simulink model "Plant_N_LQR"  (R2017a)
settings: Solver=ode5  StartTime=0.0  StopTime=t  FixedStep=0.001  RelTol=1e-3  EnableMultiTasking=on
values from neighbouring files (symbols this model uses):
  K_LQR = -R1\B'*P    [Sc_H2LQR_R.m]
  t_stop = 35    [Sc_reference.m]    (also in pathdes.m = 50)
libraries: simulink x6
settings Model: Creator=GeoLee  LastModifiedBy=gmh_n
settings DataIOCC: LimitDataPoints=on  SaveFormat=Array
settings OptimizationCC: LifeSpan=inf
settings DebuggingCC: SFUnexpectedBacktrackingDiag=warning  SFNoUnconditionalDefaultTransitionDiag=warning  SFExecutionAtInitializationDiag=none
settings HardwareCC: ProdBitPerPointer=32  ProdBitPerSizeT=32  ProdBitPerPtrDiffT=32  ProdLargestAtomicFloat=None  ProdIntDivRoundTo=Undefined  ProdEndianess=Unspecified  ProdWordSize=32  ProdHWDeviceType=32-bit Generic
settings ModelReferenceCC: PropagateSignalLabelsOutOfModel=off
settings GRTTargetCC: TargetLangStandard=C89/C90 (ANSI)  GeneratePreprocessorConditionals=Disable all
settings ConfigComp: CovMetricSettings=dw  CovHtmlReporting=on  CovSaveCumulativeToWorkspaceVar=on  CovSaveSingleToWorkspaceVar=on  CovExternalEMLEnable=off

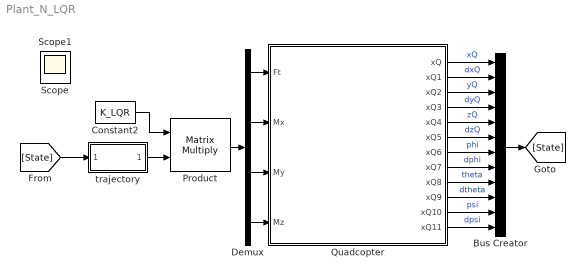
== system Plant_N_LQR ==
  Bus Creator : BusCreator  Inputs=12
  Constant2 : Constant  Value=K_LQR
  Demux : Demux
  Product : Product  Multiplication=Matrix(*)  RndMeth=Zero
  Quadcopter : Subsystem  mask(Single Quadcopter Plant){x0=0, y0=0, z0=0}
      mask prompts: x0 "Initial position of x (m)"; y0 "Initial position of y (m)"; z0 "Initial position of z (m)"
      mask help:
      | Attention:
      | the first input Ft is actually dF!
      mask Display:
      | image('Quad_pic.png');
      | port_label('input', 1, 'Ft');
      | port_label('input', 2, 'Mx');
      | port_label('input', 3, 'My');
      | port_label('input', 4, 'Mz');
      | port_label('output', 1, 'xQ');
      | port_label('output', 2, 'dxQ');
      | port_label('output', 3, 'yQ');
      | port_label('output', 4, 'dyQ');
      | port_label('output', 5, 'zQ');
      | port_label('output', 6, 'dzQ');
      | port_label('output', 7, 'phi');
      | port_label('output', 8, 'dphi');
      | port_label('output', 9, 'theta');
      | port_label('output', 10, 'dtheta');
      | port_label('output', 11, 'psi');
      | port_label('output', 12, 'dpsi');
  trajectory : Subsystem
  Scope : Scope
  Scope1 : Scope
  wires:
  Product/1 -> Demux/1
  [State] -> trajectory/1(State)
  trajectory/1(error) -> Product/2
  Quadcopter/6(xQ5) -> Bus Creator/6  "dzQ"
  Quadcopter/5(xQ4) -> Bus Creator/5  "zQ"
  Quadcopter/7(xQ6) -> Bus Creator/7  "phi"
  Quadcopter/4(xQ3) -> Bus Creator/4  "dyQ"
  Quadcopter/8(xQ7) -> Bus Creator/8  "dphi"
  Quadcopter/3(xQ2) -> Bus Creator/3  "yQ"
  Quadcopter/9(xQ8) -> Bus Creator/9  "theta"
  Quadcopter/2(xQ1) -> Bus Creator/2  "dxQ"
  Quadcopter/10(xQ9) -> Bus Creator/10  "dtheta"
  Quadcopter/11(xQ10) -> Bus Creator/11  "psi"
  Quadcopter/1(xQ) -> Bus Creator/1  "xQ"
  Quadcopter/12(xQ11) -> Bus Creator/12  "dpsi"
  Bus Creator/1 -> [State]
  Demux/1 -> Quadcopter/1(Ft)
  Demux/2 -> Quadcopter/2(Mx)
  Demux/4 -> Quadcopter/4(Mz)
  Demux/3 -> Quadcopter/3(My)
  Constant2/1 -> Product/1

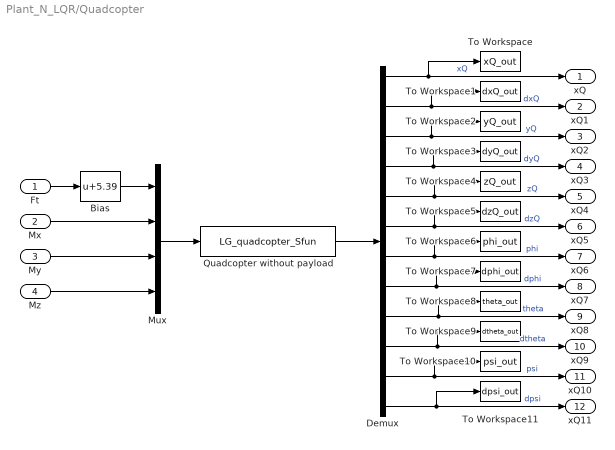
== system Plant_N_LQR/Quadcopter ==
  Ft : Inport
  Mx : Inport  Port=2
  My : Inport  Port=3
  Mz : Inport  Port=4
  Bias : Bias  Bias=5.39
  Demux : Demux  Outputs=12
  Mux : Mux
  Quadcopter without payload : S-Function  FunctionName=LG_quadcopter_Sfun  Parameters=x0,y0,z0  SFunctionDeploymentMode=off  EnableBusSupport=off
  To Workspace : ToWorkspace  VariableName=xQ_out  SampleTime=-1
  To Workspace1 : ToWorkspace  VariableName=dxQ_out  SampleTime=-1
  To Workspace10 : ToWorkspace  VariableName=psi_out  SampleTime=-1
  To Workspace11 : ToWorkspace  VariableName=dpsi_out  SampleTime=-1
  To Workspace2 : ToWorkspace  VariableName=yQ_out  SampleTime=-1
  To Workspace3 : ToWorkspace  VariableName=dyQ_out  SampleTime=-1
  To Workspace4 : ToWorkspace  VariableName=zQ_out  SampleTime=-1
  To Workspace5 : ToWorkspace  VariableName=dzQ_out  SampleTime=-1
  To Workspace6 : ToWorkspace  VariableName=phi_out  SampleTime=-1
  To Workspace7 : ToWorkspace  VariableName=dphi_out  SampleTime=-1
  To Workspace8 : ToWorkspace  VariableName=theta_out  SampleTime=-1
  To Workspace9 : ToWorkspace  VariableName=dtheta_out  SampleTime=-1
  xQ : Outport
  xQ1 : Outport  Port=2
  xQ2 : Outport  Port=3
  xQ3 : Outport  Port=4
  xQ4 : Outport  Port=5
  xQ5 : Outport  Port=6
  xQ6 : Outport  Port=7
  xQ7 : Outport  Port=8
  xQ8 : Outport  Port=9
  xQ9 : Outport  Port=10
  xQ10 : Outport  Port=11
  xQ11 : Outport  Port=12
  wires:
  Mux/1 -> Quadcopter without payload/1
  Ft/1 -> Bias/1
  Quadcopter without payload/1 -> Demux/1
  Mz/1 -> Mux/4
  Bias/1 -> Mux/1
  Demux/9 -> To Workspace8/1, xQ8/1  "theta"
  Demux/1 -> xQ/1, To Workspace/1  "xQ"
  Demux/7 -> xQ6/1, To Workspace6/1  "phi"
  Demux/11 -> xQ10/1, To Workspace10/1  "psi"
  Demux/4 -> xQ3/1, To Workspace3/1  "dyQ"
  Demux/2 -> xQ1/1, To Workspace1/1  "dxQ"
  Demux/3 -> xQ2/1, To Workspace2/1  "yQ"
  Demux/10 -> xQ9/1, To Workspace9/1  "dtheta"
  Demux/5 -> xQ4/1, To Workspace4/1  "zQ"
  Demux/8 -> xQ7/1, To Workspace7/1  "dphi"
  Demux/12 -> xQ11/1, To Workspace11/1  "dpsi"
  Demux/6 -> xQ5/1, To Workspace5/1  "dzQ"
  My/1 -> Mux/3
  Mx/1 -> Mux/2

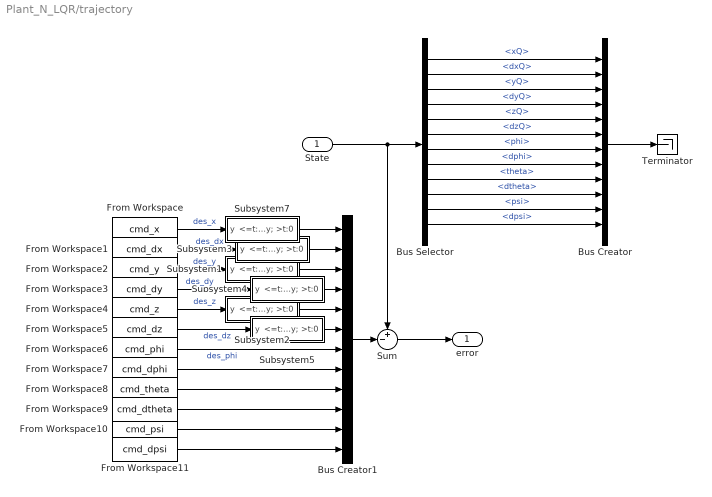
== system Plant_N_LQR/trajectory ==
  State : Inport
  Bus Creator : BusCreator  Inputs=12
  Bus Creator1 : BusCreator  Inputs=12
  Bus Selector : BusSelector  OutputSignals=xQ,dxQ,yQ,dyQ,zQ,dzQ,phi,dphi,theta,dtheta,psi,dpsi
  From Workspace : FromWorkspace  VariableName=cmd_x  SampleTime=0
  From Workspace1 : FromWorkspace  VariableName=cmd_dx  SampleTime=0
  From Workspace10 : FromWorkspace  VariableName=cmd_psi  SampleTime=0
  From Workspace11 : FromWorkspace  VariableName=cmd_dpsi  SampleTime=0
  From Workspace2 : FromWorkspace  VariableName=cmd_y  SampleTime=0
  From Workspace3 : FromWorkspace  VariableName=cmd_dy  SampleTime=0
  From Workspace4 : FromWorkspace  VariableName=cmd_z  SampleTime=0
  From Workspace5 : FromWorkspace  VariableName=cmd_dz  SampleTime=0
  From Workspace6 : FromWorkspace  VariableName=cmd_phi  SampleTime=0
  From Workspace7 : FromWorkspace  VariableName=cmd_dphi  SampleTime=0
  From Workspace8 : FromWorkspace  VariableName=cmd_theta  SampleTime=0
  From Workspace9 : FromWorkspace  VariableName=cmd_dtheta  SampleTime=0
  Subsystem1 : Subsystem
  Subsystem2 : Subsystem
  Subsystem3 : Subsystem
  Subsystem4 : Subsystem
  Subsystem5 : Subsystem
  Subsystem7 : Subsystem
  Sum : Sum  Inputs=+-|
  Terminator : Terminator
  error : Outport
  wires:
  Bus Selector/3 -> Bus Creator/3  "<yQ>"
  Bus Selector/9 -> Bus Creator/9  "<theta>"
  Bus Selector/10 -> Bus Creator/10  "<dtheta>"
  Bus Selector/7 -> Bus Creator/7  "<phi>"
  Bus Selector/2 -> Bus Creator/2  "<dxQ>"
  Bus Selector/8 -> Bus Creator/8  "<dphi>"
  Bus Selector/5 -> Bus Creator/5  "<zQ>"
  Bus Selector/4 -> Bus Creator/4  "<dyQ>"
  Bus Selector/11 -> Bus Creator/11  "<psi>"
  Bus Creator/1 -> Terminator/1
  Bus Selector/12 -> Bus Creator/12  "<dpsi>"
  Bus Selector/1 -> Bus Creator/1  "<xQ>"
  State/1 -> Bus Selector/1, Sum/1
  Bus Selector/6 -> Bus Creator/6  "<dzQ>"
  Bus Creator1/1 -> Sum/2
  From Workspace/1 -> Subsystem7/1(y)  "des_x"
  From Workspace1/1 -> Subsystem3/1(y)  "des_dx"
  From Workspace2/1 -> Subsystem1/1(y)  "des_y"
  From Workspace3/1 -> Subsystem4/1(y)  "des_dy"
  From Workspace4/1 -> Subsystem2/1(y)  "des_z"
  Sum/1 -> error/1
  From Workspace9/1 -> Bus Creator1/10
  From Workspace11/1 -> Bus Creator1/12
  From Workspace10/1 -> Bus Creator1/11
  From Workspace8/1 -> Bus Creator1/9
  From Workspace5/1 -> Subsystem5/1(y)  "des_dz"
  From Workspace6/1 -> Bus Creator1/7  "des_phi"
  From Workspace7/1 -> Bus Creator1/8
  Subsystem7/1(<=t:y; >t:0) -> Bus Creator1/1
  Subsystem1/1(<=t:y; >t:0) -> Bus Creator1/3
  Subsystem2/1(<=t:y; >t:0) -> Bus Creator1/5
  Subsystem3/1(<=t:y; >t:0) -> Bus Creator1/2
  Subsystem4/1(<=t:y; >t:0) -> Bus Creator1/4
  Subsystem5/1(<=t:y; >t:0) -> Bus Creator1/6

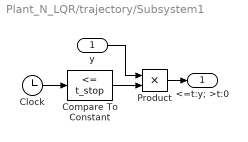
== system Plant_N_LQR/trajectory/Subsystem1 ==
  y : Inport
  Clock : Clock
  Compare To Constant : simulink/Logic and Bit Operations/Compare To Constant  relop=<=  const=t_stop  OutDataTypeStr=boolean
  Product : Product
  <=t:y; >t:0 : Outport
  wires:
  Compare To Constant/1 -> Product/2
  Product/1 -> <=t:y; >t:0/1
  y/1 -> Product/1
  Clock/1 -> Compare To Constant/1

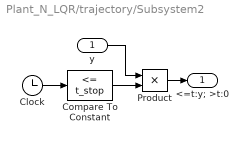
== system Plant_N_LQR/trajectory/Subsystem2 ==
  y : Inport
  Clock : Clock
  Compare To Constant : simulink/Logic and Bit Operations/Compare To Constant  relop=<=  const=t_stop  OutDataTypeStr=boolean
  Product : Product
  <=t:y; >t:0 : Outport
  wires:
  Clock/1 -> Compare To Constant/1
  y/1 -> Product/1
  Product/1 -> <=t:y; >t:0/1
  Compare To Constant/1 -> Product/2

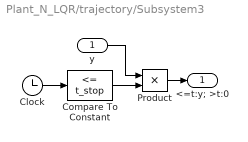
== system Plant_N_LQR/trajectory/Subsystem3 ==
  y : Inport
  Clock : Clock
  Compare To Constant : simulink/Logic and Bit Operations/Compare To Constant  relop=<=  const=t_stop  OutDataTypeStr=boolean
  Product : Product
  <=t:y; >t:0 : Outport
  wires:
  Compare To Constant/1 -> Product/2
  Product/1 -> <=t:y; >t:0/1
  y/1 -> Product/1
  Clock/1 -> Compare To Constant/1

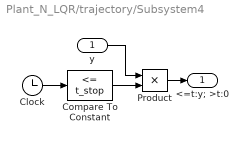
== system Plant_N_LQR/trajectory/Subsystem4 ==
  y : Inport
  Clock : Clock
  Compare To Constant : simulink/Logic and Bit Operations/Compare To Constant  relop=<=  const=t_stop  OutDataTypeStr=boolean
  Product : Product
  <=t:y; >t:0 : Outport
  wires:
  Clock/1 -> Compare To Constant/1
  y/1 -> Product/1
  Product/1 -> <=t:y; >t:0/1
  Compare To Constant/1 -> Product/2

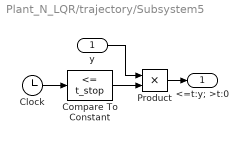
== system Plant_N_LQR/trajectory/Subsystem5 ==
  y : Inport
  Clock : Clock
  Compare To Constant : simulink/Logic and Bit Operations/Compare To Constant  relop=<=  const=t_stop  OutDataTypeStr=boolean
  Product : Product
  <=t:y; >t:0 : Outport
  wires:
  Compare To Constant/1 -> Product/2
  Product/1 -> <=t:y; >t:0/1
  y/1 -> Product/1
  Clock/1 -> Compare To Constant/1

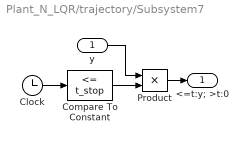
== system Plant_N_LQR/trajectory/Subsystem7 ==
  y : Inport
  Clock : Clock
  Compare To Constant : simulink/Logic and Bit Operations/Compare To Constant  relop=<=  const=t_stop  OutDataTypeStr=boolean
  Product : Product
  <=t:y; >t:0 : Outport
  wires:
  Clock/1 -> Compare To Constant/1
  y/1 -> Product/1
  Product/1 -> <=t:y; >t:0/1
  Compare To Constant/1 -> Product/2
